simulink model "lab2"  (R2012b)
settings: Solver=ode1  StartTime=0.0  StopTime=100  FixedStep=0.005  RelTol=1e-3
libraries: simulink x12
Description:
  | Created by MapleSim.
settings Model: ExtModeTrigDuration=10000  Creator=MapleSim  LastModifiedBy=artem
settings SolverCC: PositivePriorityOrder=on
settings DataIOCC: SignalLoggingSaveFormat=ModelDataLogs  SignalLogging=off  DSMLogging=off
settings OptimizationCC: InitFltsAndDblsToZero=on
settings DebuggingCC: SaveWithParameterizedLinksMsg=none  MultiTaskDSMMsg=warning  MultiTaskCondExecSysMsg=none  FcnCallInpInsideContextMsg=UseLocalSettings  StrictBusMsg=None
settings HardwareCC: TargetHWDeviceType=32-bit Generic
settings SFSimCC: SimParseCustomCode=off
settings RTWCC: SystemTargetFile=quarc_win64.tlc  TemplateMakefile=quarc_default_tmf  Description=QUARC Win64 Target  ProcessScript=quarc_win64_make_rtw_hook  IncludeERTFirstTime=on
settings CodeAppCC: CustomSymbolStrType=$N$R$M_T  InternalIdentifier=Shortened
settings STFCustomTargetCC: TargetPreCompLibLocation=C:\PROGRA~3\QUARC\lib\2011b\win64\release  CodeReplacementLibrary=ANSI_C  GeneratePreprocessorConditionals=Disable all  SystemTargetFile=quarc_win64.tlc
settings GRTTargetCC: TargetPreCompLibLocation=C:\PROGRA~3\QUARC\lib\2011b\win64\release  ParMdlRefBuildCompliant=off  CompOptLevelCompliant=off  ConcurrentExecutionCompliant=off  CombineOutputUpdateFcns=off  MatFileLogging=off  GRTInterface=on  ExtMode=on  ExtModeMexFile=quarc_comm
settings ConfigurationSet: Description=SimMechanics 2G

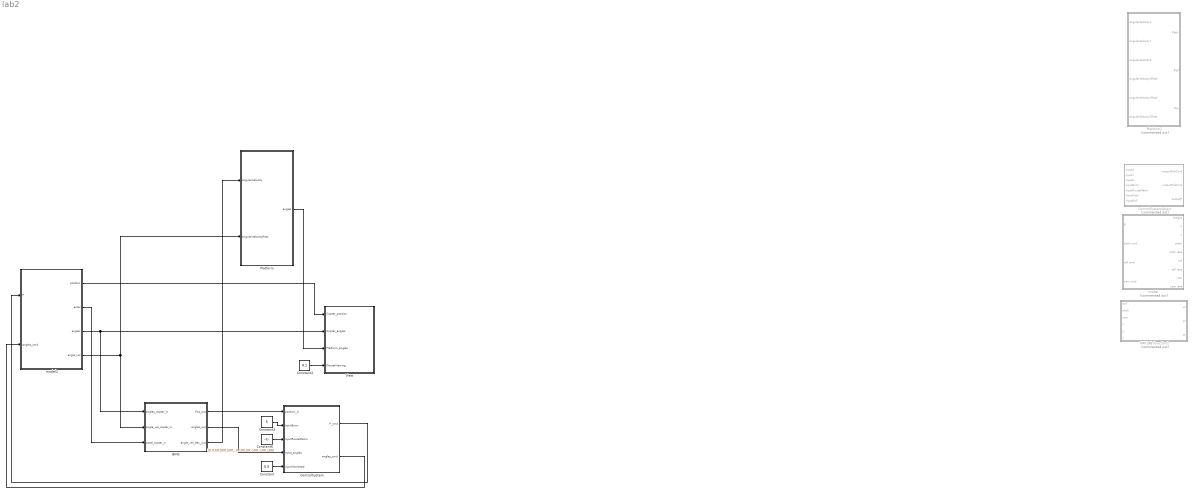
== system lab2 ==
  BINS : Subsystem
  Constant : Constant  Value=0.5
  Constant2 : Constant  Value=0.1
  Constant3 : Constant  Value=5
  Constant6 : Constant  Value=[0,0,50;500,500,50;0,20,50;100,0,50;-30,0,50;100,100,50;-100,-100,100]  VectorParams1D=off
      settings: SamplingMode=Frame based
  ControlSystem : Subsystem
  ControlSystemOrigin : Subsystem  Commented=on
  MATLAB Function2 : MATLAB Function  Commented=on  TreatAsAtomicUnit=on
  Platform : Subsystem
  Platform1 : Subsystem  Commented=on
  View : Subsystem
  model : Subsystem  Commented=on
  model2 : Subsystem
  wires:
  Constant3/1 -> ControlSystem/2(inputError)
  Constant6/1 -> ControlSystem/3(inputRouteMatrix)
  ControlSystem/1(P_cmd) -> model2/1(P)
  Constant2/1 -> View/4(DiscretViewing)
  model2/4(angle_vel) -> BINS/2(angle_vel_copter_in), Platform/2(angularVelocityReal)
  Constant/1 -> ControlSystem/5(inputYawNeed)
  Platform/1(angles) -> View/3(Platform_angles)
  model2/3(angles) -> View/2(Copter_angles), BINS/1(angles_copter_in)
  model2/2("accel ") -> BINS/3(accel_copter_in)
  BINS/1(Pos_out) -> ControlSystem/1("position_in ")
  BINS/2(angles_out) -> ControlSystem/4(input_angles)
  BINS/3(angle_vel_Nav_out) -> Platform/1(angularVelocity)
  ControlSystem/2(angles_cmd) -> model2/2(angles_cmd)
  model2/1("position ") -> View/1(Copter_position)

== system lab2/BINS ==
  angles_copter_in : Inport
  angle_vel_copter_in : Inport  Port=2
  accel_copter_in : Inport  Port=3
  AccellerIntegr : Subsystem
  Accellerometr : Subsystem
  AngularVelocitySensor : Subsystem
  Pos_out : Outport
  angles_out : Outport  Port=2
  angle_vel_Nav_out : Outport  Port=3
  wires:
  AngularVelocitySensor/1(angle_vel_Nav_out) -> AccellerIntegr/1(angle_vel_in), angle_vel_Nav_out/1
  angles_copter_in/1 -> Accellerometr/1(angles)
  angle_vel_copter_in/1 -> AngularVelocitySensor/1(angle_vel_in)
  accel_copter_in/1 -> Accellerometr/2(accel_In)
  Accellerometr/1(accel_out) -> AccellerIntegr/2(accel_in)
  AccellerIntegr/1(position_out) -> Pos_out/1
  AccellerIntegr/2(angles_out) -> angles_out/1

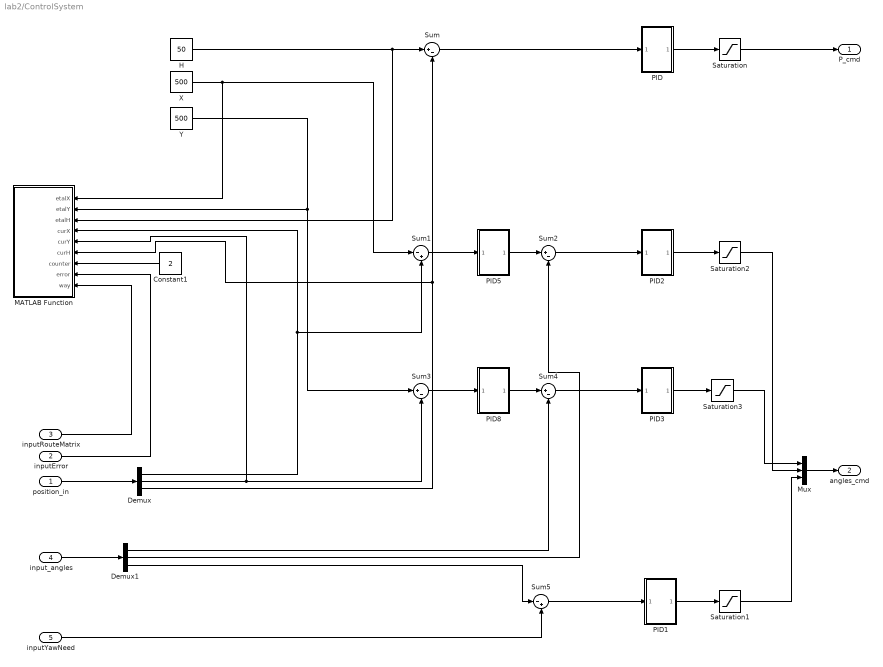
== system lab2/ControlSystem ==
  "position_in " : Inport
  inputError : Inport  Port=2
  inputRouteMatrix : Inport  Port=3
  input_angles : Inport  Port=4
  inputYawNeed : Inport  Port=5
  Constant1 : Constant  InitFcn=|  Value=2
      | coder.extrinsic('set_param');                                    
      | set_param('lab2_next_level/ControlSystem/Constant1','Value','0');
  Demux : Demux  Outputs=3
  Demux1 : Demux  Outputs=3
  H : Constant  InitFcn=|  Value=50
      | coder.extrinsic('set_param');                            
      | set_param('lab2_next_level/ControlSystem/H','Value','0');
  MATLAB Function : MATLAB Function  TreatAsAtomicUnit=on
  Mux : Mux  Inputs=3
  PID : Subsystem
  PID1 : Subsystem
  PID2 : Subsystem
  PID3 : Subsystem
  PID5 : Subsystem
  PID8 : Subsystem
  Saturation : Saturate  UpperLimit=0.1  LowerLimit=0
  Saturation1 : Saturate  UpperLimit=0.1  LowerLimit=-0.1
  Saturation2 : Saturate  UpperLimit=0.1  LowerLimit=-0.1
  Saturation3 : Saturate  UpperLimit=0.1  LowerLimit=-0.1
  Sum{,2..4} (4 alike) : Sum  Inputs=|+-
  Sum1 : Sum  Inputs=|-+
  Sum5 : Sum  Inputs=|-+
  X : Constant  InitFcn=|  Value=500
      | coder.extrinsic('set_param');                            
      | set_param('lab2_next_level/ControlSystem/X','Value','0');
  Y : Constant  InitFcn=|  Value=500
      | coder.extrinsic('set_param');                            
      | set_param('lab2_next_level/ControlSystem/Y','Value','0');
  P_cmd : Outport
  angles_cmd : Outport  Port=2
  wires:
  Saturation2/1 -> Mux/2
  PID3/1(Out1) -> Saturation3/1
  Demux/1 -> Sum1/2, MATLAB Function/4(curX)
  Saturation3/1 -> Mux/1
  PID/1(Out1) -> Saturation/1
  Saturation/1 -> P_cmd/1
  Constant1/1 -> MATLAB Function/7(counter)
  Demux1/2 -> Sum2/2
  H/1 -> Sum/1, MATLAB Function/3(etalH)
  inputRouteMatrix/1 -> MATLAB Function/9(way)
  Demux1/1 -> Sum4/2
  Sum3/1 -> PID8/1(In1)
  X/1 -> Sum1/1, MATLAB Function/1(etalX)
  Y/1 -> Sum3/1, MATLAB Function/2(etalY)
  inputError/1 -> MATLAB Function/8(error)
  Demux/2 -> MATLAB Function/5(curY), Sum3/2
  Sum/1 -> PID/1(In1)
  Demux/3 -> MATLAB Function/6(curH), Sum/2
  PID2/1(Out1) -> Saturation2/1
  Sum1/1 -> PID5/1(In1)
  Sum2/1 -> PID2/1(In1)
  Sum4/1 -> PID3/1(In1)
  PID5/1(Out1) -> Sum2/1
  PID8/1(Out1) -> Sum4/1
  PID1/1(Out1) -> Saturation1/1
  Demux1/3 -> Sum5/1
  inputYawNeed/1 -> Sum5/2
  Sum5/1 -> PID1/1(In1)
  "position_in "/1 -> Demux/1
  Saturation1/1 -> Mux/3
  Mux/1 -> angles_cmd/1
  input_angles/1 -> Demux1/1

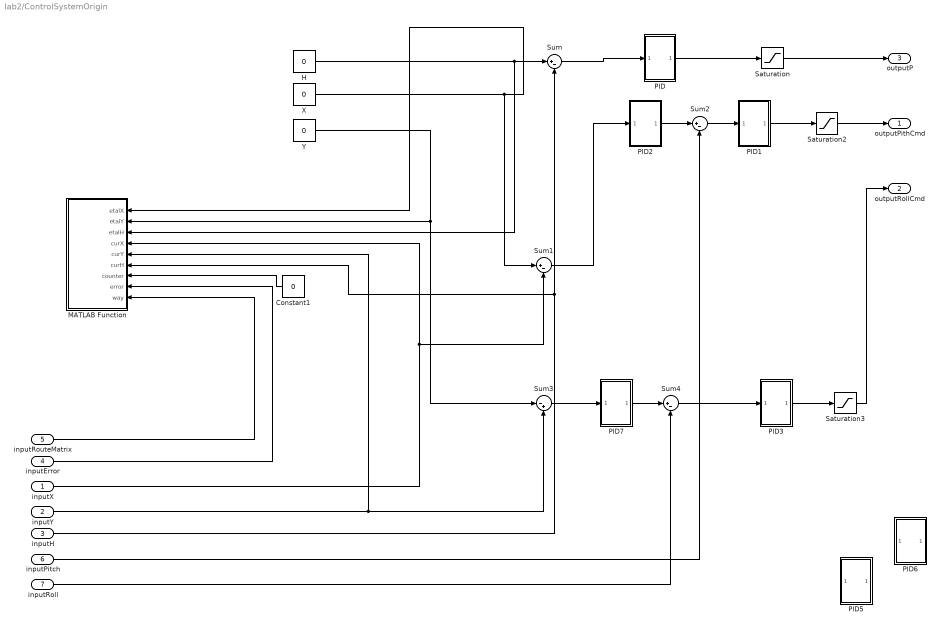
== system lab2/ControlSystemOrigin ==
  inputX : Inport
  inputY : Inport  Port=2
  inputH : Inport  Port=3
  inputError : Inport  Port=4
  inputRouteMatrix : Inport  Port=5
  inputPitch : Inport  Port=6
  inputRoll : Inport  Port=7
  Constant1 : Constant  InitFcn=|  Value=0
      | coder.extrinsic('set_param');                                    
      | set_param('lab2_next_level/ControlSystem/Constant1','Value','0');
  H : Constant  InitFcn=|  Value=0
      | coder.extrinsic('set_param');                            
      | set_param('lab2_next_level/ControlSystem/H','Value','0');
  MATLAB Function : MATLAB Function  TreatAsAtomicUnit=on
  PID : Subsystem
  PID1 : Subsystem
  PID2 : Subsystem
  PID3 : Subsystem
  PID5 : Subsystem
  PID6 : Subsystem
  PID7 : Subsystem
  Saturation : Saturate  UpperLimit=0.1  LowerLimit=0
  Saturation2 : Saturate  UpperLimit=0.1  LowerLimit=-0.1
  Saturation3 : Saturate  UpperLimit=0.01  LowerLimit=-0.01
  Sum{,1..2,4} (4 alike) : Sum  Inputs=|+-
  Sum3 : Sum  Inputs=|-+
  X : Constant  InitFcn=|  Value=0
      | coder.extrinsic('set_param');                            
      | set_param('lab2_next_level/ControlSystem/X','Value','0');
  Y : Constant  InitFcn=|  Value=0
      | coder.extrinsic('set_param');                            
      | set_param('lab2_next_level/ControlSystem/Y','Value','0');
  outputPithCmd : Outport
  outputRollCmd : Outport  Port=2
  outputP : Outport  Port=3
  wires:
  Saturation2/1 -> outputPithCmd/1
  PID3/1(Out1) -> Saturation3/1
  inputX/1 -> Sum1/2, MATLAB Function/4(curX)
  Saturation3/1 -> outputRollCmd/1
  PID/1(Out1) -> Saturation/1
  Saturation/1 -> outputP/1
  Constant1/1 -> MATLAB Function/7(counter)
  inputPitch/1 -> Sum2/2
  H/1 -> Sum/1, MATLAB Function/3(etalH)
  inputRouteMatrix/1 -> MATLAB Function/9(way)
  inputRoll/1 -> Sum4/2
  Sum3/1 -> PID7/1(In1)
  X/1 -> Sum1/1, MATLAB Function/1(etalX)
  Y/1 -> Sum3/1, MATLAB Function/2(etalY)
  inputError/1 -> MATLAB Function/8(error)
  inputY/1 -> Sum3/2, MATLAB Function/5(curY)
  Sum/1 -> PID/1(In1)
  inputH/1 -> MATLAB Function/6(curH), Sum/2
  PID1/1(Out1) -> Saturation2/1
  Sum1/1 -> PID2/1(In1)
  Sum2/1 -> PID1/1(In1)
  Sum4/1 -> PID3/1(In1)
  PID2/1(Out1) -> Sum2/1
  PID7/1(Out1) -> Sum4/1

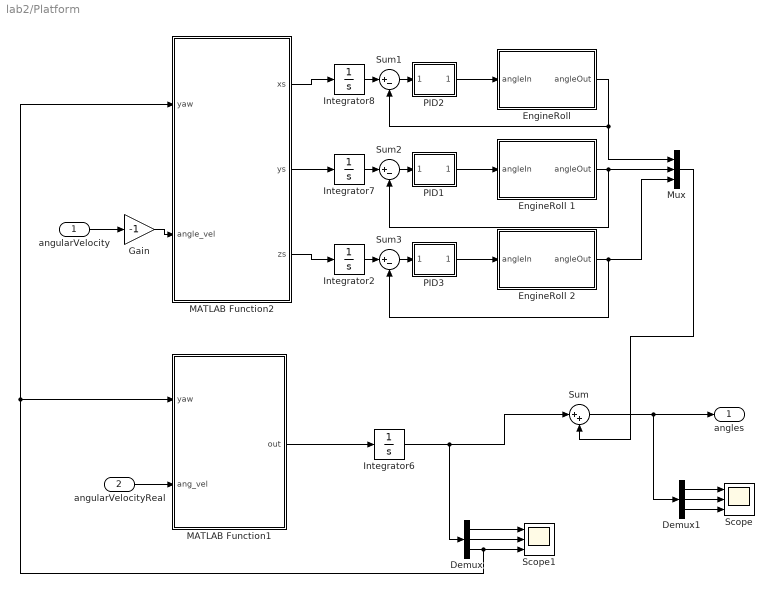
== system lab2/Platform ==
  angularVelocity : Inport
  angularVelocityReal : Inport  Port=2
  Demux : Demux  Outputs=3
  Demux1 : Demux  Outputs=3
  "EngineRoll " : Subsystem
  EngineRoll 1 : Subsystem
  EngineRoll 2 : Subsystem
  Gain : Gain  Gain=-1
  Integrator{2,6..8} (4 alike) : Integrator  LimitOutput=on  UpperSaturationLimit=1  LowerSaturationLimit=-1
  MATLAB Function1 : MATLAB Function  TreatAsAtomicUnit=on
  MATLAB Function2 : MATLAB Function  TreatAsAtomicUnit=on
  Mux : Mux  Inputs=3
  PID1 : Subsystem
  PID2 : Subsystem
  PID3 : Subsystem
  Scope : Scope  NumInputPorts=3
      settings: YMin=-0.0075~-0.02~-0.001  YMax=0.0375~0.0075~0.018  MaxDataPoints=50000000
  Scope1 : Scope  NumInputPorts=3
      settings: YMin=-0.1~-0.17~0  YMax=0.5~0.01~0.6  MaxDataPoints=50000000
  Sum : Sum  Inputs=|++
  Sum1 : Sum  Inputs=|+-
  Sum2 : Sum  Inputs=|+-
  Sum3 : Sum  Inputs=|+-
  angles : Outport
  wires:
  MATLAB Function2/3(zs) -> Integrator2/1
  MATLAB Function2/1(xs) -> Integrator8/1
  MATLAB Function2/2(ys) -> Integrator7/1
  Gain/1 -> MATLAB Function2/2(angle_vel)
  Integrator6/1 -> Sum/1, Demux/1
  Demux/3 -> MATLAB Function2/1(yaw), MATLAB Function1/1(yaw), Scope1/3
  MATLAB Function1/1(out) -> Integrator6/1
  angularVelocity/1 -> Gain/1
  angularVelocityReal/1 -> MATLAB Function1/2(ang_vel)
  Mux/1 -> Sum/2
  Sum/1 -> angles/1, Demux1/1
  Demux1/1 -> Scope/1
  Demux1/2 -> Scope/2
  Demux1/3 -> Scope/3
  Demux/1 -> Scope1/1
  Demux/2 -> Scope1/2
  "EngineRoll "/1(angleOut) -> Sum1/2, Mux/1
  PID2/1(Out1) -> "EngineRoll "/1(angleIn)
  Integrator8/1 -> Sum1/1
  Sum1/1 -> PID2/1(In1)
  EngineRoll 1/1(angleOut) -> Sum2/2, Mux/2
  PID1/1(Out1) -> EngineRoll 1/1(angleIn)
  Sum2/1 -> PID1/1(In1)
  Integrator7/1 -> Sum2/1
  EngineRoll 2/1(angleOut) -> Mux/3, Sum3/2
  PID3/1(Out1) -> EngineRoll 2/1(angleIn)
  Sum3/1 -> PID3/1(In1)
  Integrator2/1 -> Sum3/1

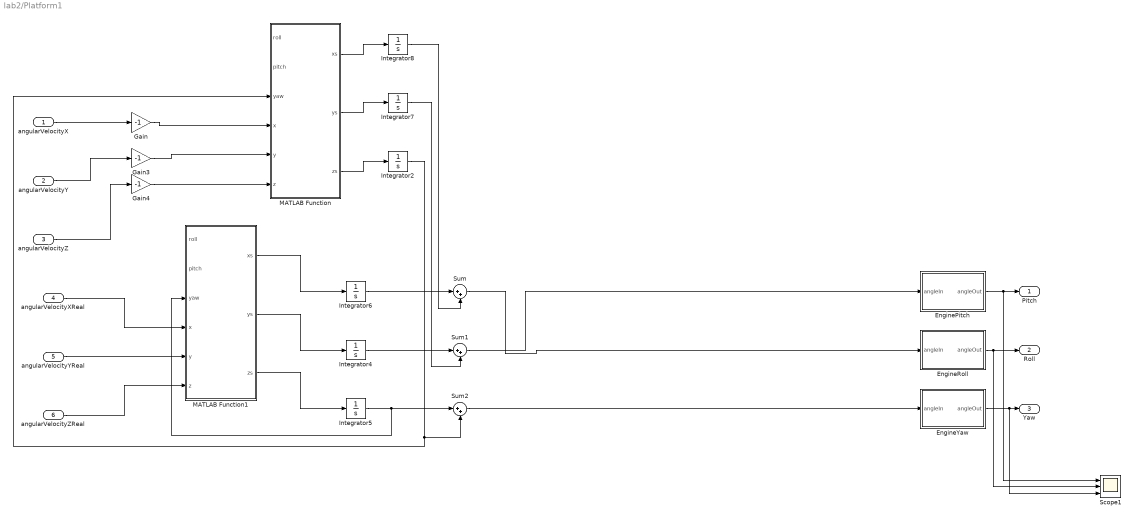
== system lab2/Platform1 ==
  angularVelocityX : Inport
  angularVelocityY : Inport  Port=2
  angularVelocityZ : Inport  Port=3
  angularVelocityXReal : Inport  Port=4
  angularVelocityYReal : Inport  Port=5
  angularVelocityZReal : Inport  Port=6
  EnginePitch : Subsystem
  EngineRoll : Subsystem
  EngineYaw : Subsystem
  Gain : Gain  Gain=-1
  Gain3 : Gain  Gain=-1
  Gain4 : Gain  Gain=-1
  Integrator{2,4..8} (6 alike) : Integrator  LimitOutput=on  UpperSaturationLimit=1  LowerSaturationLimit=-1
  MATLAB Function : MATLAB Function  TreatAsAtomicUnit=on
  MATLAB Function1 : MATLAB Function  TreatAsAtomicUnit=on
  Scope1 : Scope  NumInputPorts=3
      settings: TimeRange=10  YMin=-0.02~-0.08~0.5725  YMax=0.12~0.09~0.5925  SaveName=ScopeData4
  Sum : Sum  Inputs=|++
  Sum1 : Sum  Inputs=|++
  Sum2 : Sum  Inputs=|++
  Pitch : Outport
  Roll : Outport  Port=2
  Yaw : Outport  Port=3
  wires:
  Integrator7/1 -> Sum1/2
  Integrator2/1 -> Sum2/2, MATLAB Function/3(yaw)
  MATLAB Function/3(zs) -> Integrator2/1
  Integrator8/1 -> Sum/2
  MATLAB Function/1(xs) -> Integrator8/1
  MATLAB Function/2(ys) -> Integrator7/1
  Gain/1 -> MATLAB Function/4(x)
  Gain3/1 -> MATLAB Function/5(y)
  Gain4/1 -> MATLAB Function/6(z)
  Integrator6/1 -> Sum/1
  Integrator4/1 -> Sum1/1
  Integrator5/1 -> MATLAB Function1/3(yaw), Sum2/1
  Sum/1 -> EngineRoll/1(angleIn)
  Sum1/1 -> EnginePitch/1(angleIn)
  MATLAB Function1/1(xs) -> Integrator6/1
  MATLAB Function1/2(ys) -> Integrator4/1
  MATLAB Function1/3(zs) -> Integrator5/1
  angularVelocityX/1 -> Gain/1
  angularVelocityY/1 -> Gain3/1
  angularVelocityZ/1 -> Gain4/1
  angularVelocityXReal/1 -> MATLAB Function1/4(x)
  angularVelocityYReal/1 -> MATLAB Function1/5(y)
  angularVelocityZReal/1 -> MATLAB Function1/6(z)
  EngineRoll/1(angleOut) -> Scope1/2, Roll/1
  EngineYaw/1(angleOut) -> Scope1/3, Yaw/1
  EnginePitch/1(angleOut) -> Scope1/1, Pitch/1
  Sum2/1 -> EngineYaw/1(angleIn)

== system lab2/View ==
  Copter_position : Inport
  Copter_angles : Inport  Port=2
  Platform_angles : Inport  Port=3
  DiscretViewing : Inport  Port=4
  Clock : Clock
  Demux : Demux  Outputs=3
  Demux1 : Demux  Outputs=3
  Demux2 : Demux  Outputs=3
  Math Function : Math  Operator=mod  SaturateOnIntegerOverflow=on
  Visualisation : MATLAB Function  TreatAsAtomicUnit=on
  wires:
  DiscretViewing/1 -> Math Function/2
  Math Function/1 -> Visualisation/10(C)
  Clock/1 -> Math Function/1
  Demux2/3 -> Visualisation/6(yaw)
  Copter_position/1 -> Demux1/1
  Demux2/2 -> Visualisation/5(pitch)
  Demux2/1 -> Visualisation/4(roll)
  Demux1/2 -> Visualisation/2(y)
  Demux1/1 -> Visualisation/1(x)
  Demux/3 -> Visualisation/9(pyaw)
  Demux/2 -> Visualisation/8(ppitch)
  Demux/1 -> Visualisation/7(proll)
  Platform_angles/1 -> Demux/1
  Demux1/3 -> Visualisation/3(z)
  Copter_angles/1 -> Demux2/1

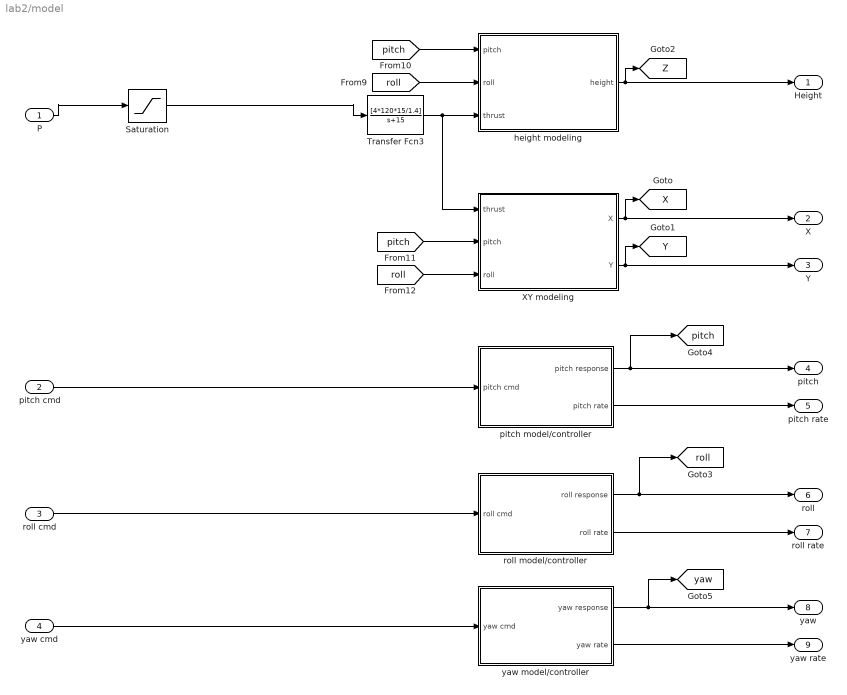
== system lab2/model ==
  P : Inport
  pitch cmd : Inport  Port=2
  roll cmd : Inport  Port=3
  yaw cmd : Inport  Port=4
  Saturation : Saturate  UpperLimit=0.1  LowerLimit=0
  Transfer Fcn3 : TransferFcn  Numerator=[4*120*15/1.4]  Denominator=[1 15]
  XY modeling : Subsystem
  height modeling : Subsystem
  pitch model/controller : Subsystem
  roll model/controller : Subsystem
  yaw model/controller : Subsystem
  "Height " : Outport
  "X " : Outport  Port=2
  "Y " : Outport  Port=3
  pitch : Outport  Port=4
  pitch rate : Outport  Port=5
  roll : Outport  Port=6
  roll rate : Outport  Port=7
  yaw : Outport  Port=8
  yaw rate : Outport  Port=9
  tag scope: X=global, Y=global, Z=global, pitch=global, roll=global, yaw=global
  wires:
  yaw cmd/1 -> yaw model/controller/1(yaw cmd)
  roll cmd/1 -> roll model/controller/1(roll cmd)
  pitch cmd/1 -> pitch model/controller/1(pitch cmd)
  P/1 -> Saturation/1
  yaw model/controller/2(yaw rate) -> yaw rate/1
  roll model/controller/2(roll rate) -> roll rate/1
  pitch model/controller/2(pitch rate) -> pitch rate/1
  XY modeling/2(Y) -> "Y "/1, [Y]
  XY modeling/1(X) -> "X "/1, [X]
  [roll] -> XY modeling/3(roll)
  [pitch] -> XY modeling/2(pitch)
  Transfer Fcn3/1 -> XY modeling/1(thrust), height modeling/3(thrust)
  [roll] -> height modeling/2(roll)
  [pitch] -> height modeling/1(pitch)
  height modeling/1(height) -> "Height "/1, [Z]
  yaw model/controller/1(yaw response) -> yaw/1, [yaw]
  roll model/controller/1(roll response) -> roll/1, [roll]
  pitch model/controller/1(pitch response) -> [pitch], pitch/1
  Saturation/1 -> Transfer Fcn3/1

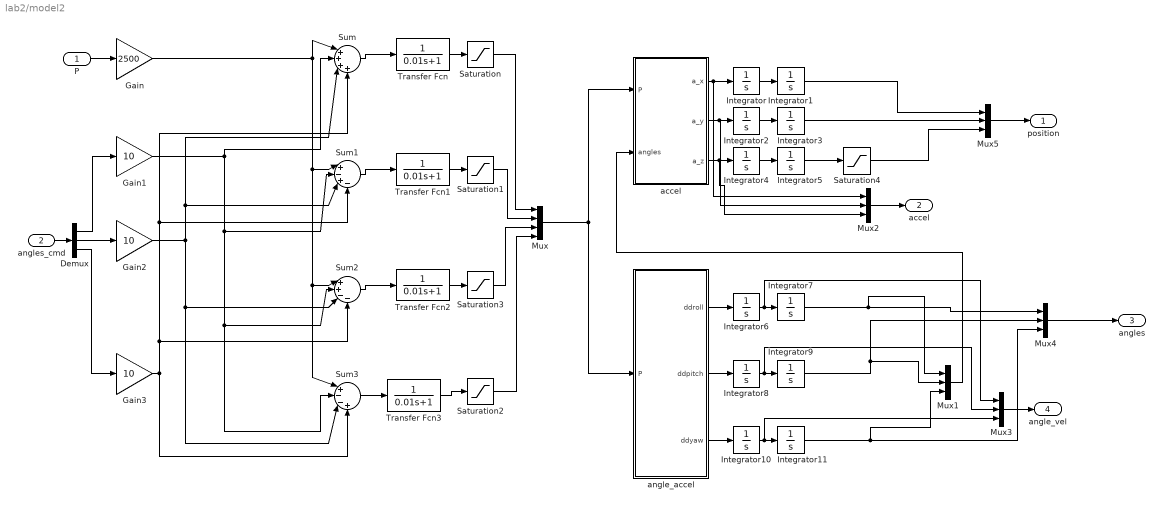
== system lab2/model2 ==
  P : Inport
  angles_cmd : Inport  Port=2
  Demux : Demux  Outputs=3
  Gain : Gain  Gain=2500
  Gain1 : Gain  Gain=10
  Gain2 : Gain  Gain=10
  Gain3 : Gain  Gain=10
  Integrator{,1..5,10..11} (8 alike) : Integrator
  Integrator{6..9} (4 alike) : Integrator  LimitOutput=on  UpperSaturationLimit=1  LowerSaturationLimit=-1
  Mux : Mux
  Mux{1..5} (5 alike) : Mux  Inputs=3
  Saturation{,1..3} (4 alike) : Saturate  UpperLimit=500  LowerLimit=0
  Saturation4 : Saturate  UpperLimit=100000000  LowerLimit=0
  Sum : Sum  Inputs=|++++
  Sum1 : Sum  Inputs=|+-+-
  Sum2 : Sum  Inputs=|++--
  Sum3 : Sum  Inputs=|+--+
  Transfer Fcn{,1..3} (4 alike) : TransferFcn  Denominator=[0.01 1]
  accel : MATLAB Function  TreatAsAtomicUnit=on
  angle_accel : MATLAB Function  TreatAsAtomicUnit=on
  "position " : Outport
  "accel " : Outport  Port=2
  angles : Outport  Port=3
  angle_vel : Outport  Port=4
  wires:
  P/1 -> Gain/1
  Gain/1 -> Sum1/1, Sum3/1, Sum2/1, Sum/1
  Sum/1 -> Transfer Fcn/1
  Sum1/1 -> Transfer Fcn1/1
  Sum2/1 -> Transfer Fcn2/1
  Sum3/1 -> Transfer Fcn3/1
  Transfer Fcn/1 -> Saturation/1
  Mux/1 -> accel/1(P), angle_accel/1(P)
  Integrator/1 -> Integrator1/1
  Integrator2/1 -> Integrator3/1
  Integrator4/1 -> Integrator5/1
  accel/1(a_x) -> Mux2/1, Integrator/1
  accel/2(a_y) -> Mux2/2, Integrator2/1
  Integrator1/1 -> Mux5/1
  Integrator3/1 -> Mux5/2
  Integrator5/1 -> Saturation4/1
  angle_accel/1(ddroll) -> Integrator6/1
  Integrator6/1 -> Mux3/1, Integrator7/1
  angle_accel/3(ddyaw) -> Integrator10/1
  angle_accel/2(ddpitch) -> Integrator8/1
  Integrator8/1 -> Mux3/2, Integrator9/1
  Integrator10/1 -> Mux3/3, Integrator11/1
  Saturation/1 -> Mux/1
  Transfer Fcn1/1 -> Saturation1/1
  Saturation1/1 -> Mux/2
  Saturation2/1 -> Mux/4
  Transfer Fcn2/1 -> Saturation3/1
  Saturation3/1 -> Mux/3
  Demux/3 -> Gain3/1
  Saturation4/1 -> Mux5/3
  Integrator7/1 -> Mux4/1, Mux1/1
  Integrator9/1 -> Mux4/2, Mux1/2
  Demux/1 -> Gain1/1
  Demux/2 -> Gain2/1
  Integrator11/1 -> Mux4/3, Mux1/3
  Mux1/1 -> accel/2(angles)
  Gain1/1 -> Sum2/2, Sum3/2, Sum1/2, Sum/2
  Gain2/1 -> Sum1/3, Sum/3, Sum2/3, Sum3/3
  Gain3/1 -> Sum2/4, Sum1/4, Sum/4, Sum3/4
  Transfer Fcn3/1 -> Saturation2/1
  Mux2/1 -> "accel "/1
  accel/3(a_z) -> Mux2/3, Integrator4/1
  Mux3/1 -> angle_vel/1
  Mux4/1 -> angles/1
  Mux5/1 -> "position "/1
  angles_cmd/1 -> Demux/1

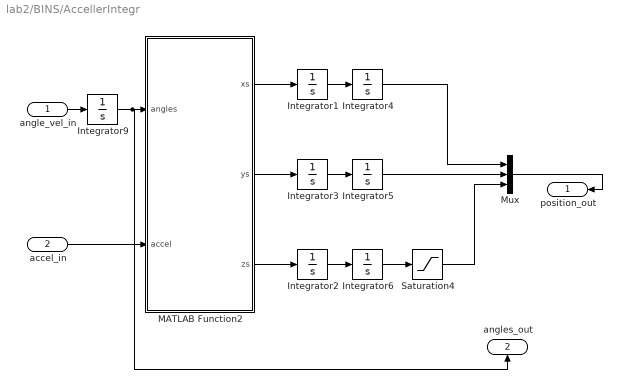
== system lab2/BINS/AccellerIntegr ==
  angle_vel_in : Inport
  accel_in : Inport  Port=2
  Integrator{1..6} (6 alike) : Integrator
  Integrator9 : Integrator  LimitOutput=on  UpperSaturationLimit=1  LowerSaturationLimit=-1
  MATLAB Function2 : MATLAB Function  TreatAsAtomicUnit=on
  Mux : Mux  Inputs=3
  Saturation4 : Saturate  UpperLimit=100000000  LowerLimit=0
  position_out : Outport
  angles_out : Outport  Port=2
  wires:
  accel_in/1 -> MATLAB Function2/2(accel)
  angle_vel_in/1 -> Integrator9/1
  MATLAB Function2/1(xs) -> Integrator1/1
  MATLAB Function2/2(ys) -> Integrator3/1
  MATLAB Function2/3(zs) -> Integrator2/1
  Integrator1/1 -> Integrator4/1
  Integrator3/1 -> Integrator5/1
  Integrator2/1 -> Integrator6/1
  Integrator4/1 -> Mux/1
  Integrator6/1 -> Saturation4/1
  Integrator9/1 -> angles_out/1, MATLAB Function2/1(angles)
  Mux/1 -> position_out/1
  Integrator5/1 -> Mux/2
  Saturation4/1 -> Mux/3

== system lab2/BINS/Accellerometr ==
  angles : Inport
  accel_In : Inport  Port=2
  MATLAB Function2 : MATLAB Function  TreatAsAtomicUnit=on
  Mux : Mux  Inputs=3
  Scope : Scope  NumInputPorts=3
      settings: YMin=-0.0025~-1~-0.00125  YMax=0.0015~1~0.00125  SaveName=ScopeData2  MaxDataPoints=50000000
  Sum : Sum  Inputs=|+-
  Sum1 : Sum  Inputs=|+-
  Transfer Fcn : TransferFcn  Denominator=[0.005 0.1]
  "WhiteNoiseVector " : Subsystem
  accel_out : Outport
  wires:
  accel_In/1 -> MATLAB Function2/2(accel)
  angles/1 -> MATLAB Function2/1(angles)
  MATLAB Function2/2(ys) -> "WhiteNoiseVector "/2(In2)
  MATLAB Function2/3(zs) -> "WhiteNoiseVector "/3(In3)
  "WhiteNoiseVector "/2(Out2) -> Mux/2
  "WhiteNoiseVector "/3(Out3) -> Mux/3
  Mux/1 -> accel_out/1
  MATLAB Function2/1(xs) -> Sum1/1, Sum/1, "WhiteNoiseVector "/1(In1)
  "WhiteNoiseVector "/1(Out1) -> Sum1/2, Mux/1, Sum/2
  Sum/1 -> Scope/3
  Sum1/1 -> Scope/1

== system lab2/BINS/AngularVelocitySensor ==
  angle_vel_in : Inport
  Demux : Demux  Outputs=3
  Mux : Mux  Inputs=3
  Rate Transition : RateTransition
  Scope : Scope  NumInputPorts=4
      settings: YMin=-0.1~-0.15~-0.0008~-0.15  YMax=0.35~0.4~0.0008~0.075  SaveName=ScopeData3  MaxDataPoints=50000
  Sum : Sum  Inputs=|+-
  Sum1 : Sum  Inputs=|+-
  Transfer Fcn : TransferFcn  Denominator=[0.2 1]  AbsoluteTolerance=1
  "WhiteNoiseVector " : Subsystem
  angle_vel_Nav_out : Outport
  wires:
  "WhiteNoiseVector "/1(Out1) -> Rate Transition/1, Mux/1, Sum/1, Scope/2
  "WhiteNoiseVector "/2(Out2) -> Mux/2
  "WhiteNoiseVector "/3(Out3) -> Mux/3
  Mux/1 -> angle_vel_Nav_out/1
  angle_vel_in/1 -> Demux/1
  Demux/1 -> Sum1/2, Sum/2, "WhiteNoiseVector "/1(In1)
  Demux/2 -> "WhiteNoiseVector "/2(In2)
  Demux/3 -> "WhiteNoiseVector "/3(In3)
  Transfer Fcn/1 -> Sum1/1, Scope/1
  Sum/1 -> Scope/3
  Sum1/1 -> Scope/4
  Rate Transition/1 -> Transfer Fcn/1

== system lab2/ControlSystem/PID ==
  In1 : Inport
  Derivative : Derivative
  Gain : Gain  Gain=0.007
  Gain1 : Gain  Gain=0.0006
  Gain2 : Gain  Gain=0.02
  Gain3 : Gain
  Integrator : Integrator
  Sum1 : Sum  Inputs=|+++
  Out1 : Outport
  wires:
  Gain1/1 -> Integrator/1
  Gain3/1 -> Sum1/1
  Integrator/1 -> Sum1/2
  Gain/1 -> Gain3/1
  In1/1 -> Gain1/1, Gain/1, Gain2/1
  Derivative/1 -> Sum1/3
  Gain2/1 -> Derivative/1
  Sum1/1 -> Out1/1

== system lab2/ControlSystem/PID1 ==
  In1 : Inport
  Derivative : Derivative
  Gain : Gain  Gain=0.012
  Gain1 : Gain  Gain=0.00048
  Gain2 : Gain  Gain=0.075
  Gain3 : Gain
  Integrator : Integrator
  Sum1 : Sum  Inputs=|+++
  Out1 : Outport
  wires:
  Gain1/1 -> Integrator/1
  Gain3/1 -> Sum1/1
  Integrator/1 -> Sum1/2
  Gain/1 -> Gain3/1
  In1/1 -> Gain1/1, Gain/1, Gain2/1
  Derivative/1 -> Sum1/3
  Gain2/1 -> Derivative/1
  Sum1/1 -> Out1/1

== system lab2/ControlSystem/PID2 ==
  In1 : Inport
  Derivative : Derivative
  Gain : Gain  Gain=0.01
  Gain1 : Gain  Gain=1e-9
  Gain2 : Gain  Gain=0.2
  Gain3 : Gain
  Integrator : Integrator
  Sum1 : Sum  Inputs=|+++
  Out1 : Outport
  wires:
  Gain1/1 -> Integrator/1
  Gain3/1 -> Sum1/1
  Integrator/1 -> Sum1/2
  Gain/1 -> Gain3/1
  In1/1 -> Gain1/1, Gain/1, Gain2/1
  Derivative/1 -> Sum1/3
  Gain2/1 -> Derivative/1
  Sum1/1 -> Out1/1

== system lab2/ControlSystem/PID3 ==
  In1 : Inport
  Derivative : Derivative
  Gain : Gain  Gain=0.01
  Gain1 : Gain  Gain=1e-9
  Gain2 : Gain  Gain=0.2
  Gain3 : Gain
  Integrator : Integrator
  Sum1 : Sum  Inputs=|+++
  Out1 : Outport
  wires:
  Gain1/1 -> Integrator/1
  Gain3/1 -> Sum1/1
  Integrator/1 -> Sum1/2
  Gain/1 -> Gain3/1
  In1/1 -> Gain1/1, Gain/1, Gain2/1
  Derivative/1 -> Sum1/3
  Gain2/1 -> Derivative/1
  Sum1/1 -> Out1/1

== system lab2/ControlSystem/PID5 ==
  In1 : Inport
  Derivative : Derivative
  Gain : Gain  Gain=0.02
  Gain1 : Gain  Gain=1e-9
  Gain2 : Gain  Gain=0.15
  Gain3 : Gain
  Integrator : Integrator
  Sum1 : Sum  Inputs=|+++
  Out1 : Outport
  wires:
  Gain1/1 -> Integrator/1
  Gain3/1 -> Sum1/1
  Integrator/1 -> Sum1/2
  Gain/1 -> Gain3/1
  In1/1 -> Gain1/1, Gain/1, Gain2/1
  Derivative/1 -> Sum1/3
  Gain2/1 -> Derivative/1
  Sum1/1 -> Out1/1

== system lab2/ControlSystem/PID8 ==
  In1 : Inport
  Derivative : Derivative
  Gain : Gain  Gain=0.02
  Gain1 : Gain  Gain=1e-9
  Gain2 : Gain  Gain=0.15
  Gain3 : Gain
  Integrator : Integrator
  Sum1 : Sum  Inputs=|+++
  Out1 : Outport
  wires:
  Gain1/1 -> Integrator/1
  Gain3/1 -> Sum1/1
  Integrator/1 -> Sum1/2
  Gain/1 -> Gain3/1
  In1/1 -> Gain1/1, Gain/1, Gain2/1
  Derivative/1 -> Sum1/3
  Gain2/1 -> Derivative/1
  Sum1/1 -> Out1/1

== system lab2/ControlSystemOrigin/PID ==
  In1 : Inport
  Derivative : Derivative
  Gain : Gain  Gain=0.006
  Gain1 : Gain  Gain=3.831578947e-04
  Gain2 : Gain  Gain=0.0361325
  Gain3 : Gain
  Integrator : Integrator
  Sum1 : Sum  Inputs=|+++
  Out1 : Outport
  wires:
  Gain1/1 -> Integrator/1
  Gain3/1 -> Sum1/1
  Integrator/1 -> Sum1/2
  Gain/1 -> Gain3/1
  In1/1 -> Gain1/1, Gain/1, Gain2/1
  Derivative/1 -> Sum1/3
  Gain2/1 -> Derivative/1
  Sum1/1 -> Out1/1

== system lab2/ControlSystemOrigin/PID1 ==
  In1 : Inport
  Derivative : Derivative
  Gain : Gain  Gain=6e-03
  Gain1 : Gain  Gain=6e-9
  Gain2 : Gain  Gain=0.0255
  Gain3 : Gain
  Integrator : Integrator
  Sum1 : Sum  Inputs=|+++
  Out1 : Outport
  wires:
  Gain1/1 -> Integrator/1
  Gain3/1 -> Sum1/1
  Integrator/1 -> Sum1/2
  Gain/1 -> Gain3/1
  In1/1 -> Gain1/1, Gain/1, Gain2/1
  Derivative/1 -> Sum1/3
  Gain2/1 -> Derivative/1
  Sum1/1 -> Out1/1

== system lab2/ControlSystemOrigin/PID2 ==
  In1 : Inport
  Derivative : Derivative
  Gain : Gain  Gain=0.010
  Gain1 : Gain  Gain=7.058823529e-09
  Gain2 : Gain  Gain=0.141875
  Gain3 : Gain
  Integrator : Integrator
  Sum1 : Sum  Inputs=|+++
  Out1 : Outport
  wires:
  Gain1/1 -> Integrator/1
  Gain3/1 -> Sum1/1
  Integrator/1 -> Sum1/2
  Gain/1 -> Gain3/1
  In1/1 -> Gain1/1, Gain/1, Gain2/1
  Derivative/1 -> Sum1/3
  Gain2/1 -> Derivative/1
  Sum1/1 -> Out1/1

== system lab2/ControlSystemOrigin/PID3 ==
  In1 : Inport
  Derivative : Derivative
  Gain : Gain  Gain=5e-03
  Gain1 : Gain  Gain=6e-9
  Gain2 : Gain  Gain=0.035
  Gain3 : Gain
  Integrator : Integrator
  Sum1 : Sum  Inputs=|+++
  Out1 : Outport
  wires:
  Gain1/1 -> Integrator/1
  Gain3/1 -> Sum1/1
  Integrator/1 -> Sum1/2
  Gain/1 -> Gain3/1
  In1/1 -> Gain1/1, Gain/1, Gain2/1
  Derivative/1 -> Sum1/3
  Gain2/1 -> Derivative/1
  Sum1/1 -> Out1/1

== system lab2/ControlSystemOrigin/PID5 ==
  In1 : Inport
  Derivative : Derivative
  Gain : Gain  Gain=0.0005
  Gain1 : Gain  Gain=2e-09
  Gain2 : Gain  Gain=0.0545
  Gain3 : Gain
  Integrator : Integrator
  Sum1 : Sum  Inputs=|+++
  Out1 : Outport
  wires:
  Gain1/1 -> Integrator/1
  Gain3/1 -> Sum1/1
  Integrator/1 -> Sum1/2
  Gain/1 -> Gain3/1
  In1/1 -> Gain1/1, Gain/1, Gain2/1
  Derivative/1 -> Sum1/3
  Gain2/1 -> Derivative/1
  Sum1/1 -> Out1/1

== system lab2/ControlSystemOrigin/PID6 ==
  In1 : Inport
  Derivative : Derivative
  Gain : Gain  Gain=1e-03
  Gain1 : Gain  Gain=2.4e-07
  Gain2 : Gain  Gain=9e-05
  Gain3 : Gain
  Integrator : Integrator
  Sum1 : Sum  Inputs=|+++
  Out1 : Outport
  wires:
  Gain1/1 -> Integrator/1
  Gain3/1 -> Sum1/1
  Integrator/1 -> Sum1/2
  Gain/1 -> Gain3/1
  In1/1 -> Gain1/1, Gain2/1, Gain/1
  Derivative/1 -> Sum1/3
  Gain2/1 -> Derivative/1
  Sum1/1 -> Out1/1

== system lab2/ControlSystemOrigin/PID7 ==
  In1 : Inport
  Derivative : Derivative
  Gain : Gain  Gain=0.013
  Gain1 : Gain  Gain=7.058823529e-08
  Gain2 : Gain  Gain=0.171875
  Gain3 : Gain
  Integrator : Integrator
  Sum1 : Sum  Inputs=|+++
  Out1 : Outport
  wires:
  Gain1/1 -> Integrator/1
  Gain3/1 -> Sum1/1
  Integrator/1 -> Sum1/2
  Gain/1 -> Gain3/1
  In1/1 -> Gain1/1, Gain/1, Gain2/1
  Derivative/1 -> Sum1/3
  Gain2/1 -> Derivative/1
  Sum1/1 -> Out1/1

== system lab2/Platform/EngineRoll  ==
  angleIn : Inport
  Band-Limited White Noise2 : simulink/Sources/Band-Limited White Noise  Cov=[0.00001]  Ts=0.1  seed=[23341]
  Gain : Gain  Gain=10
  Integrator1 : Integrator
  Rate Transition : RateTransition
  Sum : Sum  Inputs=|+-
  Sum2 : Sum  Inputs=|++
  Transfer Fcn : TransferFcn  Denominator=[1 1]
  angleOut : Outport
  wires:
  Gain/1 -> Transfer Fcn/1
  Rate Transition/1 -> Sum2/2
  Band-Limited White Noise2/1 -> Rate Transition/1
  Transfer Fcn/1 -> Sum2/1
  Sum2/1 -> Integrator1/1
  Integrator1/1 -> angleOut/1
  angleIn/1 -> Sum/1
  Sum/1 -> Gain/1

== system lab2/Platform/EngineRoll 1 ==
  angleIn : Inport
  Band-Limited White Noise2 : simulink/Sources/Band-Limited White Noise  Cov=[0.00001]  Ts=0.1  seed=[23341]
  Gain : Gain  Gain=10
  Integrator1 : Integrator
  Rate Transition : RateTransition
  Sum : Sum  Inputs=|+-
  Sum2 : Sum  Inputs=|++
  Transfer Fcn : TransferFcn  Denominator=[1 1]
  angleOut : Outport
  wires:
  Gain/1 -> Transfer Fcn/1
  Rate Transition/1 -> Sum2/2
  Band-Limited White Noise2/1 -> Rate Transition/1
  Transfer Fcn/1 -> Sum2/1
  Sum2/1 -> Integrator1/1
  Integrator1/1 -> angleOut/1
  angleIn/1 -> Sum/1
  Sum/1 -> Gain/1

== system lab2/Platform/EngineRoll 2 ==
  angleIn : Inport
  Band-Limited White Noise2 : simulink/Sources/Band-Limited White Noise  Cov=[0.00001]  Ts=0.1  seed=[23341]
  Gain : Gain  Gain=10
  Integrator1 : Integrator
  Rate Transition : RateTransition
  Sum : Sum  Inputs=|+-
  Sum2 : Sum  Inputs=|++
  Transfer Fcn : TransferFcn  Denominator=[1 1]
  angleOut : Outport
  wires:
  Gain/1 -> Transfer Fcn/1
  Rate Transition/1 -> Sum2/2
  Band-Limited White Noise2/1 -> Rate Transition/1
  Transfer Fcn/1 -> Sum2/1
  Sum2/1 -> Integrator1/1
  Integrator1/1 -> angleOut/1
  angleIn/1 -> Sum/1
  Sum/1 -> Gain/1

== system lab2/Platform/PID1 ==
  In1 : Inport
  Derivative : Derivative
  Gain : Gain  Gain=0.2
  Gain1 : Gain  Gain=1e-4
  Gain3 : Gain
  Gain4 : Gain  Gain=1.65
  Integrator : Integrator
  Sum1 : Sum  Inputs=|+++
  Out1 : Outport
  wires:
  Gain1/1 -> Integrator/1
  Gain3/1 -> Sum1/1
  Integrator/1 -> Sum1/2
  Gain/1 -> Gain3/1
  In1/1 -> Gain4/1, Gain1/1, Gain/1
  Derivative/1 -> Sum1/3
  Gain4/1 -> Derivative/1
  Sum1/1 -> Out1/1

== system lab2/Platform/PID2 ==
  In1 : Inport
  Derivative : Derivative
  Gain : Gain  Gain=0.2
  Gain1 : Gain  Gain=1e-4
  Gain3 : Gain
  Gain4 : Gain  Gain=1.65
  Integrator : Integrator
  Sum1 : Sum  Inputs=|+++
  Out1 : Outport
  wires:
  Gain1/1 -> Integrator/1
  Gain3/1 -> Sum1/1
  Integrator/1 -> Sum1/2
  Gain/1 -> Gain3/1
  In1/1 -> Gain4/1, Gain1/1, Gain/1
  Derivative/1 -> Sum1/3
  Gain4/1 -> Derivative/1
  Sum1/1 -> Out1/1

== system lab2/Platform/PID3 ==
  In1 : Inport
  Derivative : Derivative
  Gain : Gain  Gain=0.2
  Gain1 : Gain  Gain=1e-4
  Gain3 : Gain
  Gain4 : Gain  Gain=1.65
  Integrator : Integrator
  Sum1 : Sum  Inputs=|+++
  Out1 : Outport
  wires:
  Gain1/1 -> Integrator/1
  Gain3/1 -> Sum1/1
  Integrator/1 -> Sum1/2
  Gain/1 -> Gain3/1
  In1/1 -> Gain4/1, Gain1/1, Gain/1
  Derivative/1 -> Sum1/3
  Gain4/1 -> Derivative/1
  Sum1/1 -> Out1/1

== system lab2/Platform1/EnginePitch ==
  angleIn : Inport
  Band-Limited White Noise2 : simulink/Sources/Band-Limited White Noise  Cov=[0.00001]  Ts=0.1  seed=[23341]
  Gain : Gain  Gain=10
  Integrator1 : Integrator
  PID2 : Subsystem
  Rate Transition : RateTransition
  Saturation : Saturate  UpperLimit=1  LowerLimit=-1
  Sum : Sum  Inputs=|+-
  Sum2 : Sum  Inputs=|++
  Transfer Fcn : TransferFcn  Denominator=[1 1]
  angleOut : Outport
  wires:
  Gain/1 -> Transfer Fcn/1
  Rate Transition/1 -> Sum2/2
  Band-Limited White Noise2/1 -> Rate Transition/1
  Transfer Fcn/1 -> Sum2/1
  Sum2/1 -> Integrator1/1
  Integrator1/1 -> angleOut/1, Sum/2
  Sum/1 -> PID2/1(In1)
  angleIn/1 -> Saturation/1
  Saturation/1 -> Sum/1
  PID2/1(Out1) -> Gain/1

== system lab2/Platform1/EngineRoll ==
  angleIn : Inport
  Band-Limited White Noise2 : simulink/Sources/Band-Limited White Noise  Cov=[0.00001]  Ts=0.1  seed=[23341]
  Gain : Gain  Gain=100
  Integrator1 : Integrator
  PID2 : Subsystem
  Rate Transition : RateTransition
  Saturation : Saturate  UpperLimit=1  LowerLimit=-1
  Sum : Sum  Inputs=|+-
  Sum2 : Sum  Inputs=|++
  Transfer Fcn : TransferFcn  Denominator=[1 1]
  angleOut : Outport
  wires:
  Gain/1 -> Transfer Fcn/1
  Rate Transition/1 -> Sum2/2
  Band-Limited White Noise2/1 -> Rate Transition/1
  Transfer Fcn/1 -> Sum2/1
  Sum2/1 -> Integrator1/1
  Integrator1/1 -> angleOut/1, Sum/2
  Sum/1 -> PID2/1(In1)
  angleIn/1 -> Saturation/1
  Saturation/1 -> Sum/1
  PID2/1(Out1) -> Gain/1

== system lab2/Platform1/EngineYaw ==
  angleIn : Inport
  Band-Limited White Noise2 : simulink/Sources/Band-Limited White Noise  Cov=[0.00001]  Ts=0.1  seed=[23341]
  Gain : Gain  Gain=10
  Integrator1 : Integrator
  PID2 : Subsystem
  Rate Transition : RateTransition
  Saturation : Saturate  UpperLimit=1  LowerLimit=-1
  Sum : Sum  Inputs=|+-
  Sum2 : Sum  Inputs=|++
  Transfer Fcn : TransferFcn  Denominator=[1 1]
  angleOut : Outport
  wires:
  Gain/1 -> Transfer Fcn/1
  Rate Transition/1 -> Sum2/2
  Band-Limited White Noise2/1 -> Rate Transition/1
  Transfer Fcn/1 -> Sum2/1
  Sum2/1 -> Integrator1/1
  Integrator1/1 -> angleOut/1, Sum/2
  Sum/1 -> PID2/1(In1)
  angleIn/1 -> Saturation/1
  Saturation/1 -> Sum/1
  PID2/1(Out1) -> Gain/1

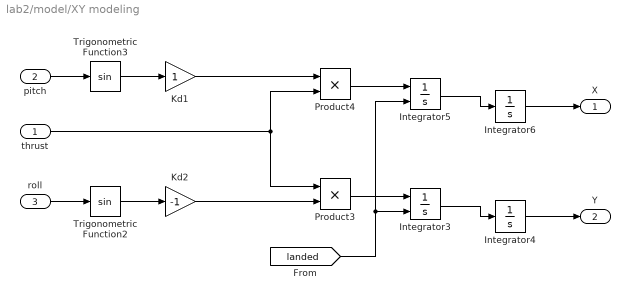
== system lab2/model/XY modeling ==
  thrust : Inport
  pitch : Inport  Port=2
  roll : Inport  Port=3
  Integrator3 : Integrator  ExternalReset=level
  Integrator4 : Integrator  LowerSaturationLimit=-0.5
  Integrator5 : Integrator  ExternalReset=level
  Integrator6 : Integrator  LowerSaturationLimit=-0.5
  Kd1 : Gain
  Kd2 : Gain  Gain=-1
  Product3 : Product  RndMeth=Zero
  Product4 : Product  RndMeth=Zero
  Trigonometric Function2 : Trigonometry
  Trigonometric Function3 : Trigonometry
  X : Outport
  Y : Outport  Port=2
  wires:
  Trigonometric Function2/1 -> Kd2/1
  Product3/1 -> Integrator3/1
  Integrator3/1 -> Integrator4/1
  Product4/1 -> Integrator5/1
  Integrator5/1 -> Integrator6/1
  Trigonometric Function3/1 -> Kd1/1
  Kd1/1 -> Product4/1
  Kd2/1 -> Product3/2
  pitch/1 -> Trigonometric Function3/1
  thrust/1 -> Product3/1, Product4/2
  roll/1 -> Trigonometric Function2/1
  Integrator4/1 -> Y/1
  Integrator6/1 -> X/1
  [landed] -> Integrator5/2, Integrator3/2

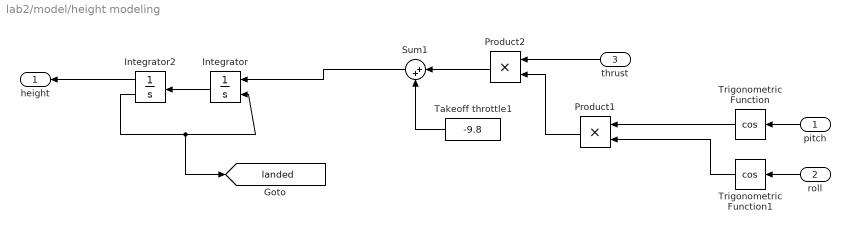
== system lab2/model/height modeling ==
  pitch : Inport
  roll : Inport  Port=2
  thrust : Inport  Port=3
  Integrator : Integrator  ExternalReset=falling
  Integrator2 : Integrator  InitialCondition=0.236  LimitOutput=on  LowerSaturationLimit=0.236  ShowSaturationPort=on
  Product1 : Product  RndMeth=Zero
  Product2 : Product  RndMeth=Zero
  Sum1 : Sum  Inputs=|++
  Takeoff throttle1 : Constant  Value=-9.8
  Trigonometric Function : Trigonometry  Operator=cos
  Trigonometric Function1 : Trigonometry  Operator=cos
  height : Outport
  tag scope: landed=global
  wires:
  Trigonometric Function/1 -> Product1/1
  Trigonometric Function1/1 -> Product1/2
  Product2/1 -> Sum1/1
  Product1/1 -> Product2/2
  Sum1/1 -> Integrator/1
  Takeoff throttle1/1 -> Sum1/2
  Integrator2/1 -> height/1
  Integrator/1 -> Integrator2/1
  thrust/1 -> Product2/1
  pitch/1 -> Trigonometric Function/1
  roll/1 -> Trigonometric Function1/1
  Integrator2/2 -> Integrator/2, [landed]

== system lab2/model/pitch model//controller ==
  pitch cmd : Inport
  pitch model : Subsystem
  pitch response : Outport
  pitch rate : Outport  Port=2
  wires:
  pitch model/2(pitch rate) -> pitch rate/1
  pitch cmd/1 -> pitch model/1(u_pitch)
  pitch model/1(pitch) -> pitch response/1

== system lab2/model/roll model//controller ==
  roll cmd : Inport
  roll model : Subsystem
  roll response : Outport
  roll rate : Outport  Port=2
  wires:
  roll model/2(roll rate) -> roll rate/1
  roll model/1(roll) -> roll response/1
  roll cmd/1 -> roll model/1(u_roll)

== system lab2/model/yaw model//controller ==
  yaw cmd : Inport
  yaw model : Subsystem
  yaw response : Outport
  yaw rate : Outport  Port=2
  wires:
  yaw model/2(yaw rate) -> yaw rate/1
  yaw cmd/1 -> yaw model/1(u_yaw)
  yaw model/1(yaw) -> yaw response/1

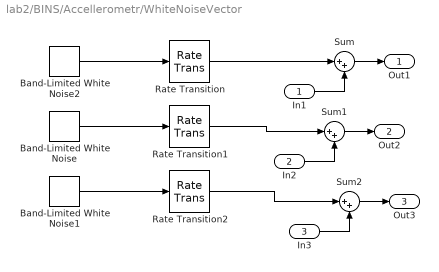
== system lab2/BINS/Accellerometr/WhiteNoiseVector  ==
  In1 : Inport
  In2 : Inport  Port=2
  In3 : Inport  Port=3
  Band-Limited White Noise : simulink/Sources/Band-Limited White Noise  Cov=[1e-8]  Ts=0.1  seed=[23341]
  Band-Limited White Noise1 : simulink/Sources/Band-Limited White Noise  Cov=[1e-8]  Ts=0.1  seed=[23341]
  Band-Limited White Noise2 : simulink/Sources/Band-Limited White Noise  Cov=[1e-8]  Ts=0.1  seed=[23341]
  Rate Transition : RateTransition
  Rate Transition1 : RateTransition
  Rate Transition2 : RateTransition
  Sum : Sum  Inputs=|++
  Sum1 : Sum  Inputs=|++
  Sum2 : Sum  Inputs=|++
  Out1 : Outport
  Out2 : Outport  Port=2
  Out3 : Outport  Port=3
  wires:
  Band-Limited White Noise2/1 -> Rate Transition/1
  Band-Limited White Noise/1 -> Rate Transition1/1
  Sum/1 -> Out1/1
  Band-Limited White Noise1/1 -> Rate Transition2/1
  In1/1 -> Sum/2
  Sum1/1 -> Out2/1
  In2/1 -> Sum1/2
  Sum2/1 -> Out3/1
  In3/1 -> Sum2/2
  Rate Transition/1 -> Sum/1
  Rate Transition1/1 -> Sum1/1
  Rate Transition2/1 -> Sum2/1

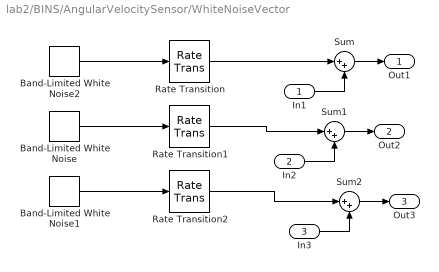
== system lab2/BINS/AngularVelocitySensor/WhiteNoiseVector  ==
  In1 : Inport
  In2 : Inport  Port=2
  In3 : Inport  Port=3
  Band-Limited White Noise : simulink/Sources/Band-Limited White Noise  Cov=[1e-8]  Ts=0.1  seed=[23341]
  Band-Limited White Noise1 : simulink/Sources/Band-Limited White Noise  Cov=[1e-8]  Ts=0.1  seed=[23341]
  Band-Limited White Noise2 : simulink/Sources/Band-Limited White Noise  Cov=[1e-8]  Ts=0.1  seed=[23341]
  Rate Transition : RateTransition
  Rate Transition1 : RateTransition
  Rate Transition2 : RateTransition
  Sum : Sum  Inputs=|++
  Sum1 : Sum  Inputs=|++
  Sum2 : Sum  Inputs=|++
  Out1 : Outport
  Out2 : Outport  Port=2
  Out3 : Outport  Port=3
  wires:
  Band-Limited White Noise2/1 -> Rate Transition/1
  Band-Limited White Noise/1 -> Rate Transition1/1
  Sum/1 -> Out1/1
  Band-Limited White Noise1/1 -> Rate Transition2/1
  In1/1 -> Sum/2
  Sum1/1 -> Out2/1
  In2/1 -> Sum1/2
  Sum2/1 -> Out3/1
  In3/1 -> Sum2/2
  Rate Transition/1 -> Sum/1
  Rate Transition1/1 -> Sum1/1
  Rate Transition2/1 -> Sum2/1

== system lab2/Platform1/EnginePitch/PID2 ==
  In1 : Inport
  Derivative : Derivative
  Gain : Gain  Gain=2
  Gain1 : Gain  Gain=7.058823529e-07
  Gain2 : Gain  Gain=0.51875
  Gain3 : Gain
  Integrator : Integrator
  Sum1 : Sum  Inputs=|+++
  Out1 : Outport
  wires:
  Gain1/1 -> Integrator/1
  Gain3/1 -> Sum1/1
  Integrator/1 -> Sum1/2
  Gain/1 -> Gain3/1
  In1/1 -> Gain1/1, Gain/1, Gain2/1
  Derivative/1 -> Sum1/3
  Gain2/1 -> Derivative/1
  Sum1/1 -> Out1/1

== system lab2/Platform1/EngineRoll/PID2 ==
  In1 : Inport
  Derivative : Derivative
  Gain : Gain  Gain=2
  Gain1 : Gain  Gain=7.058823529e-07
  Gain2 : Gain  Gain=0.51875
  Gain3 : Gain
  Integrator : Integrator
  Sum1 : Sum  Inputs=|+++
  Out1 : Outport
  wires:
  Gain1/1 -> Integrator/1
  Gain3/1 -> Sum1/1
  Integrator/1 -> Sum1/2
  Gain/1 -> Gain3/1
  In1/1 -> Gain1/1, Gain/1, Gain2/1
  Derivative/1 -> Sum1/3
  Gain2/1 -> Derivative/1
  Sum1/1 -> Out1/1

== system lab2/Platform1/EngineYaw/PID2 ==
  In1 : Inport
  Derivative : Derivative
  Gain : Gain  Gain=2
  Gain1 : Gain  Gain=7.058823529e-07
  Gain2 : Gain  Gain=0.51875
  Gain3 : Gain
  Integrator : Integrator
  Sum1 : Sum  Inputs=|+++
  Out1 : Outport
  wires:
  Gain1/1 -> Integrator/1
  Gain3/1 -> Sum1/1
  Integrator/1 -> Sum1/2
  Gain/1 -> Gain3/1
  In1/1 -> Gain1/1, Gain/1, Gain2/1
  Derivative/1 -> Sum1/3
  Gain2/1 -> Derivative/1
  Sum1/1 -> Out1/1

== system lab2/model/pitch model//controller/pitch model ==
  u_pitch : Inport
  Demux : Demux
  State-Space : StateSpace  A=[0 1 0 0; 0 0 1600 0; 0 0 -15 0; 1 0 0 0]  B=[0;0;15;0]  C=[1 0 0 0; 0 1 0 0; 0 0 1 0; 0 0 0 1]  D=[0;0;0;0]
  Terminator_1 : Terminator
  Terminator_2 : Terminator
  pitch : Outport
  pitch rate : Outport  Port=2
  wires:
  Demux/4 -> Terminator_2/1
  Demux/3 -> Terminator_1/1
  u_pitch/1 -> State-Space/1
  Demux/2 -> pitch rate/1
  Demux/1 -> pitch/1
  State-Space/1 -> Demux/1

== system lab2/model/roll model//controller/roll model ==
  u_roll : Inport
  Demux : Demux
  State-Space : StateSpace  A=[0 1 0 0; 0 0 1600 0; 0 0 -15 0; 1 0 0 0]  B=[0;0;15;0]  C=[1 0 0 0; 0 1 0 0; 0 0 1 0; 0 0 0 1]  D=[0;0;0;0]
  Terminator_1 : Terminator
  Terminator_2 : Terminator
  roll : Outport
  roll rate : Outport  Port=2
  wires:
  Demux/4 -> Terminator_2/1
  Demux/3 -> Terminator_1/1
  u_roll/1 -> State-Space/1
  Demux/2 -> roll rate/1
  Demux/1 -> roll/1
  State-Space/1 -> Demux/1

== system lab2/model/yaw model//controller/yaw model ==
  u_yaw : Inport
  Integrator5 : Integrator
  Integrator6 : Integrator  LowerSaturationLimit=-0.5
  gain : Gain  Gain=4*4/0.032
  yaw : Outport
  yaw rate : Outport  Port=2
  wires:
  u_yaw/1 -> gain/1
  Integrator6/1 -> yaw/1
  gain/1 -> Integrator5/1
  Integrator5/1 -> yaw rate/1, Integrator6/1

== matlab function lab2/ControlSystem/MATLAB Function ==
  data: etalX input; etalY input; etalH input; curX input; curY input; curH input; counter input; error input; way input
function fcn(etalX,etalY,etalH,curX,curY,curH,counter,error,way)
%#codegen
coder.extrinsic('set_param');
coder.extrinsic('num2str');

[max,el] = size(way);

if abs(etalX-curX)<=error && abs(etalY-curY)<=error && abs(etalH-curH)<=error && counter<max,
    counter = counter + 1;
    set_param('lab2_next_level/ControlSystem/Constant1','Value',num2str(counter));
    set_param('lab2_next_level/ControlSystem/X','Value',num2str(way(counter,1)));
    set_param('lab2_next_level/ControlSystem/Y','Value',num2str(way(counter,2)));
    set_param('lab2_next_level/ControlSystem/H','Value',num2str(way(counter,3)));
end;

== matlab function lab2/MATLAB Function2 ==
  data: roll input; pitch input; yaw input; x input; y input; z input; xs output; ys output; zs output
function [xs,ys,zs] = fromNavToAircraft(roll,pitch,yaw,x,y,z)
%#codegen
%from navigation to aircraft coordinate system
tr = [cos(pitch)*cos(yaw), -cos(roll)*sin(pitch)*cos(yaw)-sin(roll)*sin(yaw), sin(roll)*sin(pitch)*cos(yaw)-cos(roll)*sin(yaw);
      sin(pitch), cos(roll)*cos(pitch), -sin(roll)*cos(pitch);
      cos(pitch)*sin(yaw), -cos(roll)*sin(pitch)*sin(yaw)+sin(roll)*cos(yaw), sin(roll)*sin(pitch)*sin(yaw)+cos(roll)*cos(yaw)];
bx = [x;y;z];
ax = (tr.')*bx;

xs = ax(1);
ys = ax(2);
zs = ax(3);

== matlab function lab2/View/Visualisation ==
  data: x input; y input; z input; roll input; pitch input; yaw input; proll input; ppitch input; pyaw input; C input
function fcn(x,y,z,roll,pitch,yaw,proll,ppitch,pyaw,C)
%#codegen
coder.extrinsic('plot3')
coder.extrinsic('grid')
coder.extrinsic('axis')
coder.extrinsic('view')
coder.extrinsic('rotationMatrix');

if(C ~= 0)
    return
end

AXES = [100,0,0;0,100,0;0,0,100];

M = zeros(3,3,'double');
M = rotationMatrix(roll,pitch,yaw);
M = M*AXES;

MX = [x,M(1,1)+x;y,M(2,1)+y;z,M(3,1)+z];
MY = [x,M(1,2)+x;y,M(2,2)+y;z,M(3,2)+z];
MZ = [x,M(1,3)+x;y,M(2,3)+y;z,M(3,3)+z];

P = zeros(3,3,'double');
P = rotationMatrix(proll,ppitch,pyaw);
P = P*AXES;

PX = [x,P(1,1)+x;y,P(2,1)+y;z,P(3,1)+z];
PY = [x,P(1,2)+x;y,P(2,2)+y;z,P(3,2)+z];
PZ = [x,P(1,3)+x;y,P(2,3)+y;z,P(3,3)+z];

[az, el] = view;
plot3(x,y,z, 'or',MX(1,:),MX(2,:),MX(3,:), '-r',MY(1,:),MY(2,:),MY(3,:), '-g',MZ(1,:),MZ(2,:),MZ(3,:), '-b',PX(1,:),PX(2,:),PX(3,:), '--m',PY(1,:),PY(2,:),PY(3,:), '--k',PZ(1,:),PZ(2,:),PZ(3,:), '--c',[x+50,x+50,x-50,x-50,x+50],[y+50,y-50,y-50,y+50,y+50],[z,z,z,z,z]);
axis([-1000 1000 -1000 1000 0 500])
grid on
view([az, el]);


end

== matlab function lab2/model2/accel ==
  data: P input; a_x output; angles input; a_y output; a_z output
function [a_x, a_y, a_z] = fcn(P, angles)

roll = angles(1);
pitch = angles(2);
yaw = angles(3);

C_x = [1,0,0;
       0, cos(roll), sin(roll);
       0, -sin(roll), cos(roll)];
C_y = [cos(pitch),0,-sin(pitch);
       0, 1, 0;
       sin(pitch), 0, cos(pitch)];
C_z = [cos(yaw),sin(yaw),0;
       -sin(yaw), cos(yaw), 0;
       0, 0, 1];
   
C = C_z*C_x*C_y;

proectP = C*[0;0;1];

P_sum = sum(P);


k_x = 0.9;
k_y = 0.9;
k_z = 0.9;

m = 10;
g = 9.8;

a_x = proectP(1)*P_sum * k_x / m;

a_y = proectP(2)*P_sum * k_y / m;

a_z = proectP(3)*P_sum * k_z / m - g;

== matlab function lab2/model2/angle_accel ==
  data: P input; ddroll output; ddpitch output; ddyaw output
function [ddroll, ddpitch, ddyaw] = fcn(P)

%distance between oneside engine
h = 0.5;

Jx = 1;
Jy = 1;
Jz = 1;

M_x = (P(1)-P(2)+P(3)-P(4))*h/Jx;
M_y = (P(1)+P(2)-P(3)-P(4))*h/Jy;
k=0.5;
M_z = (P(1)+P(4)-P(2)-P(3))*h*k/Jz;

k_roll = 0.8;
k_pitch = 0.8;
k_yaw = 0.8;


ddroll = M_x * k_roll;
ddpitch = M_y * k_pitch;
ddyaw = M_z * k_yaw;

== matlab function lab2/ControlSystemOrigin/MATLAB Function ==
  data: etalX input; etalY input; etalH input; curX input; curY input; curH input; counter input; error input; way input
function fcn(etalX,etalY,etalH,curX,curY,curH,counter,error,way)
%#codegen
coder.extrinsic('set_param');
coder.extrinsic('num2str');

[max,el] = size(way);

if abs(etalX-curX)<=error && abs(etalY-curY)<=error && abs(etalH-curH)<=error && counter<max,
    counter = counter + 1;
    set_param('lab2_next_level/ControlSystem/Constant1','Value',num2str(counter));
    set_param('lab2_next_level/ControlSystem/X','Value',num2str(way(counter,1)));
    set_param('lab2_next_level/ControlSystem/Y','Value',num2str(way(counter,2)));
    set_param('lab2_next_level/ControlSystem/H','Value',num2str(way(counter,3)));
end;

== matlab function lab2/Platform/MATLAB Function2 ==
  data: yaw input; angle_vel input; xs output; ys output; zs output
function [xs,ys,zs] = fromAircraftToPlatform(yaw,angle_vel)
%#codegen
%from navigation to aircraft coordinate system

x = angle_vel(1);
y = angle_vel(2);
z = angle_vel(3);
coder.extrinsic('rotationMatrix');

ya = yaw ;
cy = cos(ya);      sy = sin(ya);

CZ = [cy,sy,0;-sy,cy,0;0,0,1];

M = CZ'*[x;y;z];

xs = M(1);
ys = M(2);
zs = M(3);

== matlab function lab2/Platform/MATLAB Function1 ==
  data: yaw input; ang_vel input; out output
function out   = fromAircraftToPlatform(yaw,ang_vel)
%#codegen
%from navigation to aircraft coordinate system

x = ang_vel(1);
y = ang_vel(2);
z = ang_vel(3);
coder.extrinsic('rotationMatrix');

ya = yaw ;
cy = cos(ya);      sy = sin(ya);

CZ = [cy,sy,0;-sy,cy,0;0,0,1];

M = CZ'*[x;y;z];

out = [0;0;0];
out(1) = M(1);
out(2) = M(2);
out(3) = M(3);

== matlab function lab2/Platform1/MATLAB Function ==
  data: roll input; pitch input; yaw input; x input; y input; z input; xs output; ys output; zs output
function [xs,ys,zs] = fromAircraftToPlatform(roll,pitch,yaw,x,y,z)
%#codegen
%from navigation to aircraft coordinate system

coder.extrinsic('rotationMatrix');
roll = 0;pitch= 0;

cr = cos(roll);     sr = sin(roll); 
cp = cos(pitch);    sp = sin(pitch);
cy = cos(yaw);      sy = sin(yaw);

CY = [cp,0,-sp;0,1,0;sp,0,cp];
CX = [1,0,0;0,cr,sr;0,-sr,cr];
CZ = [cy,sy,0;-sy,cy,0;0,0,1];

M = CZ*[x;y;z];

xs = M(1);
ys = M(2);
zs = M(3);

== matlab function lab2/Platform1/MATLAB Function1 ==
  data: roll input; pitch input; yaw input; x input; y input; z input; xs output; ys output; zs output
function [xs,ys,zs] = fromAircraftToPlatform(roll,pitch,yaw,x,y,z)
%#codegen
%from navigation to aircraft coordinate system

coder.extrinsic('rotationMatrix');
roll = 0;pitch= 0;

cr = cos(roll);     sr = sin(roll); 
cp = cos(pitch);    sp = sin(pitch);
cy = cos(yaw);      sy = sin(yaw);

CY = [cp,0,-sp;0,1,0;sp,0,cp];
CX = [1,0,0;0,cr,sr;0,-sr,cr];
CZ = [cy,sy,0;-sy,cy,0;0,0,1];

M = CZ'*[x;y;z];

xs = M(1);
ys = M(2);
zs = M(3);

== matlab function lab2/BINS/Accellerometr/MATLAB Function2 ==
  data: angles input; accel input; xs output; ys output; zs output
function [xs,ys,zs] = fromAbsToNav(angles,accel)
%#codegen
%from navigation to aircraft coordinate system

roll = angles(1);
pitch = angles(1);
yaw = angles(3);

x = accel(1);
y = accel(2);
z = accel(3);

coder.extrinsic('rotationMatrix');

P = zeros(3,3,'double');
P = rotationMatrix(roll,pitch,yaw);

M = P*[x;y;z];

xs = M(1);
ys = M(2);
zs = M(3);

== matlab function lab2/BINS/AccellerIntegr/MATLAB Function2 ==
  data: angles input; accel input; xs output; ys output; zs output
function [xs,ys,zs] = fromNavToAbs(angles,accel)
%#codegen
%from navigation to aircraft coordinate system

roll = angles(1);
pitch = angles(1);
yaw = angles(3);

x = accel(1);
y = accel(2);
z = accel(3);

coder.extrinsic('rotationMatrix');

P = zeros(3,3,'double');
P = rotationMatrix(roll,pitch,yaw);

M = P'*[x;y;z];

xs = M(1);
ys = M(2);
zs = M(3);
